simulink model "benchmark_model"  (R2021a)
settings: Solver=ode1  StartTime=0.0  StopTime=Tend  FixedStep=0.0001  MaxStep=0.1  MinStep=0.0001  AbsTol=0.01  EnableMultiTasking=on
undefined symbols (not defined in the file): A1, A2, AL, AM0, AREA, BORE, C_EGR, c_f, c_T, CAIR, cCO, cCO2, cH2, cH2O, cHC, cN2, CO, CO2, cO2, DEN0, DiscIntNeverNeededParam, EGR_dia, EGR_sk, EX_AREA, EX_M_AR, EXO, FD0, FOM, FR0, FR_C1, FR_C2, FR_C3, FR_C4, FR_C5, H2, H2O, HC, INC, INO, KET, Kex, Kh, MAS0, MCh, MHC, MN2, MO2, MOLcylT, N2, O2, PR0, R150, Rabs, SPEC, TBORE, Th_HC, Th_knock, THEX, THIN, TM0 ... (+9)
libraries: pid_lib x1
(part 5 of 6)

== system benchmark_model/ENGINE/engine_s/cylinders/cyl3/cyl/frame/Init_cyl_gas/capture_cyl_state ==
  cyl_gas : Inport
  Trigger : TriggerPort  VariantControl=(inherit)
  Add : Sum  Inputs=++++
  C+O2->CO2 : Constant  Value=4.19*97200.0
  CO+1/2O2->CO2 : Constant  Value=4.19*29620.0
  H+1/2O2->H2O : Constant  Value=4.19*57750.0
  H+1/2O2->H2O1 : Constant  Value=4.19*57750.0
  H/C : Constant  Value=y/2
  Product : Product  RndMeth=Zero
  Product1 : Product  RndMeth=Zero
  Product2 : Product  RndMeth=Zero
  Product3 : Product  Inputs=3  RndMeth=Zero
  Saturation : Saturate  UpperLimit=22  LowerLimit=6
  Selector1 : Selector  InputPortWidth=7  IndexOptions=Index vector (dialog)  Indices=[3]  OutputSizes=[(-2)]
  Selector2 : Selector  InputPortWidth=7  IndexOptions=Index vector (dialog)  Indices=[5]  OutputSizes=[(-2)]
  Selector3 : Selector  InputPortWidth=7  IndexOptions=Index vector (dialog)  Indices=[1]  OutputSizes=[(-2)]
  Selector4 : Selector  InputPortWidth=7  IndexOptions=Index vector (dialog)  Indices=[1]  OutputSizes=[(-2)]
  Subtract : Sum  Inputs=-+
  burnt_compsition : Subsystem
  cal_af : Subsystem
  Qmax : Outport
  b_comp : Outport  Port=2  InitialOutput=[0;0;0;0;0;0;0]
  init_gas : Outport  Port=3  InitialOutput=[0;0;0;0;0;0;0]
  af : Outport  Port=4  InitialOutput=0
  wires:
  Subtract/1 -> Selector3/1, Selector2/1, Selector1/1, Selector4/1
  Add/1 -> Qmax/1
  H+1/2O2->H2O/1 -> Product2/2
  Selector2/1 -> Product2/1
  CO+1/2O2->CO2/1 -> Product1/2
  Selector1/1 -> Product1/1
  C+O2->CO2/1 -> Product/2
  burnt_compsition/1(b_comp) -> b_comp/1, Subtract/1
  cal_af/1(af) -> Saturation/1, burnt_compsition/1(af)
  cyl_gas/1 -> init_gas/1, burnt_compsition/2(mol_su), Subtract/2, cal_af/1(cyl_gas)
  Product/1 -> Add/1
  Product1/1 -> Add/2
  Product2/1 -> Add/3
  H+1/2O2->H2O1/1 -> Product3/2
  Selector3/1 -> Product3/1
  Product3/1 -> Add/4
  H/C/1 -> Product3/3
  Saturation/1 -> af/1
  Selector4/1 -> Product/1

== system benchmark_model/ENGINE/engine_s/cylinders/cyl3/cyl/frame/ratio_burnt1/mod720(u,4*pi) ==
  u : Inport
  Constant7 : Constant  Value=4*pi
  Math Function : Math  Operator=mod  SignedPower=on  SaturateOnIntegerOverflow=on
  y : Outport
  wires:
  Math Function/1 -> y/1
  u/1 -> Math Function/1
  Constant7/1 -> Math Function/2

== system benchmark_model/ENGINE/engine_s/cylinders/cyl3/cyl/frame/ratio_burnt1/murnt_ratio ==
  u : Inport
  SA : Inport  Port=2
  rps : Inport  Port=3
  KL : Inport  Port=4
  AF : Inport  Port=5
  EGR : Inport  Port=6
  VT : Inport  Port=7
  Constant2 : Constant  Value=2
  Constant6 : Constant  Value=6
  Embedded MATLAB Function : MATLAB Function  TreatAsAtomicUnit=on
  Gain1 : Gain  Gain=2
  Gain2 : Gain  Gain=180/pi
  Gain3 : Gain  Gain=pi/180
  Mux : Mux
  Phi050 DoE model : Subsystem
  q : Outport
  Q : Outport  Port=2
  wires:
  Gain3/1 -> Mux/4
  Embedded MATLAB Function/1(q) -> q/1
  SA/1 -> Gain3/1, Phi050 DoE model/3(SA)
  Mux/1 -> Embedded MATLAB Function/2(Web)
  Constant6/1 -> Mux/1
  Constant2/1 -> Mux/2
  Phi050 DoE model/1(Phi50) -> Gain1/1
  rps/1 -> Phi050 DoE model/1(N)
  KL/1 -> Phi050 DoE model/2(KL)
  VT/1 -> Gain2/1
  AF/1 -> Phi050 DoE model/5(AFR)
  Gain1/1 -> Mux/3
  EGR/1 -> Phi050 DoE model/6(EGR)
  u/1 -> Embedded MATLAB Function/1(u)
  Embedded MATLAB Function/2(Q) -> Q/1
  Gain2/1 -> Phi050 DoE model/4(VVT)

== system benchmark_model/ENGINE/engine_s/cylinders/cyl3/cyl/knock_Integral/Subsystem1/Subsystem ==
  Tu : Inport
  Constant1 : Constant  Value=FR_C3
  Divide : Product  Inputs=/*
  Math Function1 : Math  SignedPower=on  SaturateOnIntegerOverflow=on
  Saturation : Saturate  UpperLimit=inf  LowerLimit=1.0e-5
  Out1 : Outport
  wires:
  Constant1/1 -> Divide/2
  Divide/1 -> Math Function1/1
  Math Function1/1 -> Out1/1
  Tu/1 -> Saturation/1
  Saturation/1 -> Divide/1

== system benchmark_model/ENGINE/engine_s/cylinders/cyl3/cyl/knock_Integral/Subsystem1/cal_unburned_temp ==
  Pc : Inport
  Tc : Inport  Port=2
  trg_inc : Inport  Port=3
  Constant : Constant  Value=1-1/Kex
  Divide3 : Product  Inputs=*/
  Divide4 : Product
  Math Function2 : Math  Operator=pow  SignedPower=on  SaturateOnIntegerOverflow=on
  Subsystem : Subsystem
  Tu : Outport
  wires:
  Subsystem/1(Pc_inc) -> Divide3/2
  Divide3/1 -> Math Function2/1
  Math Function2/1 -> Divide4/1
  Subsystem/2(Tc_inc) -> Divide4/2
  Constant/1 -> Math Function2/2
  Divide4/1 -> Tu/1
  Tc/1 -> Subsystem/2(Tc)
  Pc/1 -> Subsystem/1(Pc), Divide3/1
  trg_inc/1 -> Subsystem/Trigger

== system benchmark_model/ENGINE/engine_s/cylinders/cyl4/cyl/Energy_Int/dvol/func_d_cylvol(u,SPEC) ==
  In1 : Inport
  Constant1 : Constant  Value=SPEC
  Embedded MATLAB Function1 : MATLAB Function  TreatAsAtomicUnit=on
  Out1 : Outport
  wires:
  Embedded MATLAB Function1/1(y) -> Out1/1
  In1/1 -> Embedded MATLAB Function1/1(u)
  Constant1/1 -> Embedded MATLAB Function1/2(SPEC)

== system benchmark_model/ENGINE/engine_s/cylinders/cyl4/cyl/frame/Init_cyl_gas/capture_cyl_state ==
  cyl_gas : Inport
  Trigger : TriggerPort  VariantControl=(inherit)
  Add : Sum  Inputs=++++
  C+O2->CO2 : Constant  Value=4.19*97200.0
  CO+1/2O2->CO2 : Constant  Value=4.19*29620.0
  H+1/2O2->H2O : Constant  Value=4.19*57750.0
  H+1/2O2->H2O1 : Constant  Value=4.19*57750.0
  H/C : Constant  Value=y/2
  Product : Product  RndMeth=Zero
  Product1 : Product  RndMeth=Zero
  Product2 : Product  RndMeth=Zero
  Product3 : Product  Inputs=3  RndMeth=Zero
  Saturation : Saturate  UpperLimit=22  LowerLimit=6
  Selector1 : Selector  InputPortWidth=7  IndexOptions=Index vector (dialog)  Indices=[3]  OutputSizes=[(-2)]
  Selector2 : Selector  InputPortWidth=7  IndexOptions=Index vector (dialog)  Indices=[5]  OutputSizes=[(-2)]
  Selector3 : Selector  InputPortWidth=7  IndexOptions=Index vector (dialog)  Indices=[1]  OutputSizes=[(-2)]
  Selector4 : Selector  InputPortWidth=7  IndexOptions=Index vector (dialog)  Indices=[1]  OutputSizes=[(-2)]
  Subtract : Sum  Inputs=-+
  burnt_compsition : Subsystem
  cal_af : Subsystem
  Qmax : Outport
  b_comp : Outport  Port=2  InitialOutput=[0;0;0;0;0;0;0]
  init_gas : Outport  Port=3  InitialOutput=[0;0;0;0;0;0;0]
  af : Outport  Port=4  InitialOutput=0
  wires:
  Selector4/1 -> Product/1
  Saturation/1 -> af/1
  H/C/1 -> Product3/3
  Product3/1 -> Add/4
  Selector3/1 -> Product3/1
  H+1/2O2->H2O1/1 -> Product3/2
  Product2/1 -> Add/3
  Product1/1 -> Add/2
  Product/1 -> Add/1
  cyl_gas/1 -> cal_af/1(cyl_gas), Subtract/2, burnt_compsition/2(mol_su), init_gas/1
  cal_af/1(af) -> burnt_compsition/1(af), Saturation/1
  burnt_compsition/1(b_comp) -> Subtract/1, b_comp/1
  C+O2->CO2/1 -> Product/2
  Selector1/1 -> Product1/1
  CO+1/2O2->CO2/1 -> Product1/2
  Selector2/1 -> Product2/1
  H+1/2O2->H2O/1 -> Product2/2
  Add/1 -> Qmax/1
  Subtract/1 -> Selector4/1, Selector1/1, Selector2/1, Selector3/1

== system benchmark_model/ENGINE/engine_s/cylinders/cyl4/cyl/frame/ratio_burnt1/mod720(u,4*pi) ==
  u : Inport
  Constant7 : Constant  Value=4*pi
  Math Function : Math  Operator=mod  SignedPower=on  SaturateOnIntegerOverflow=on
  y : Outport
  wires:
  Constant7/1 -> Math Function/2
  u/1 -> Math Function/1
  Math Function/1 -> y/1

== system benchmark_model/ENGINE/engine_s/cylinders/cyl4/cyl/frame/ratio_burnt1/murnt_ratio ==
  u : Inport
  SA : Inport  Port=2
  rps : Inport  Port=3
  KL : Inport  Port=4
  AF : Inport  Port=5
  EGR : Inport  Port=6
  VT : Inport  Port=7
  Constant2 : Constant  Value=2
  Constant6 : Constant  Value=6
  Embedded MATLAB Function : MATLAB Function  TreatAsAtomicUnit=on
  Gain1 : Gain  Gain=2
  Gain2 : Gain  Gain=180/pi
  Gain3 : Gain  Gain=pi/180
  Mux : Mux
  Phi050 DoE model : Subsystem
  q : Outport
  Q : Outport  Port=2
  wires:
  Gain2/1 -> Phi050 DoE model/4(VVT)
  Embedded MATLAB Function/2(Q) -> Q/1
  u/1 -> Embedded MATLAB Function/1(u)
  EGR/1 -> Phi050 DoE model/6(EGR)
  Gain1/1 -> Mux/3
  AF/1 -> Phi050 DoE model/5(AFR)
  VT/1 -> Gain2/1
  KL/1 -> Phi050 DoE model/2(KL)
  rps/1 -> Phi050 DoE model/1(N)
  Phi050 DoE model/1(Phi50) -> Gain1/1
  Constant2/1 -> Mux/2
  Constant6/1 -> Mux/1
  Mux/1 -> Embedded MATLAB Function/2(Web)
  SA/1 -> Phi050 DoE model/3(SA), Gain3/1
  Embedded MATLAB Function/1(q) -> q/1
  Gain3/1 -> Mux/4

== system benchmark_model/ENGINE/engine_s/cylinders/cyl4/cyl/knock_Integral/Subsystem1/Subsystem ==
  Tu : Inport
  Constant1 : Constant  Value=FR_C3
  Divide : Product  Inputs=/*
  Math Function1 : Math  SignedPower=on  SaturateOnIntegerOverflow=on
  Saturation : Saturate  UpperLimit=inf  LowerLimit=1.0e-5
  Out1 : Outport
  wires:
  Saturation/1 -> Divide/1
  Tu/1 -> Saturation/1
  Math Function1/1 -> Out1/1
  Divide/1 -> Math Function1/1
  Constant1/1 -> Divide/2

== system benchmark_model/ENGINE/engine_s/cylinders/cyl4/cyl/knock_Integral/Subsystem1/cal_unburned_temp ==
  Pc : Inport
  Tc : Inport  Port=2
  trg_inc : Inport  Port=3
  Constant : Constant  Value=1-1/Kex
  Divide3 : Product  Inputs=*/
  Divide4 : Product
  Math Function2 : Math  Operator=pow  SignedPower=on  SaturateOnIntegerOverflow=on
  Subsystem : Subsystem
  Tu : Outport
  wires:
  trg_inc/1 -> Subsystem/Trigger
  Pc/1 -> Divide3/1, Subsystem/1(Pc)
  Tc/1 -> Subsystem/2(Tc)
  Divide4/1 -> Tu/1
  Constant/1 -> Math Function2/2
  Subsystem/2(Tc_inc) -> Divide4/2
  Math Function2/1 -> Divide4/1
  Divide3/1 -> Math Function2/1
  Subsystem/1(Pc_inc) -> Divide3/2

== system benchmark_model/ENGINE/engine_s/cylinders/cyl1/cyl/frame/Init_cyl_gas/capture_cyl_state/burnt_compsition ==
  af : Inport
  mol_su : Inport  Port=2
  C : Constant  Value=WOM
  C1 : Constant  Value=WOM
  Dot Product : DotProduct  InputSameDT=on  OutDataTypeStr=Inherit: Inherit via internal rule
  Dot Product2 : DotProduct  InputSameDT=on  OutDataTypeStr=Inherit: Inherit via internal rule
  Mux : Mux  Inputs=7
  Product1 : Product  RndMeth=Zero
  Product2 : Product  Inputs=/*  RndMeth=Zero
  Saturation : Saturate  UpperLimit=22  LowerLimit=6
  Subsystem : Subsystem
  table_CO : Lookup  InputValues=AL  Table=[CO]*1.0e-2
  table_CO2 : Lookup  InputValues=AL  Table=[CO2]*1.0e-2
  table_H2 : Lookup  InputValues=AL  Table=[H2]*1.0e-2
  table_H2O : Lookup  InputValues=AL  Table=[H2O]*1.0e-2
  table_HC : Lookup  InputValues=AL  Table=[HC]*1.0e-6
  table_N2 : Lookup  InputValues=AL  Table=[N2]*1.0e-2
  table_O2 : Lookup  InputValues=AL  Table=[O2]*1.0e-2
  b_comp : Outport
  wires:
  Product2/1 -> Product1/2
  Product1/1 -> Subsystem/2(burnt)
  C/1 -> Dot Product/2
  table_HC/1 -> Mux/1
  table_N2/1 -> Mux/7
  table_CO2/1 -> Mux/2
  table_CO/1 -> Mux/3
  table_O2/1 -> Mux/4
  table_H2/1 -> Mux/5
  table_H2O/1 -> Mux/6
  af/1 -> Saturation/1, Subsystem/1(af)
  Mux/1 -> Product1/1, Dot Product/1
  Saturation/1 -> table_HC/1, table_CO2/1, table_CO/1, table_O2/1, table_H2/1, table_H2O/1, table_N2/1
  mol_su/1 -> Subsystem/3(unburnt), Dot Product2/2
  Subsystem/1(Out1) -> b_comp/1
  C1/1 -> Dot Product2/1
  Dot Product/1 -> Product2/1
  Dot Product2/1 -> Product2/2

== system benchmark_model/ENGINE/engine_s/cylinders/cyl1/cyl/frame/Init_cyl_gas/capture_cyl_state/cal_af ==
  cyl_gas : Inport
  Constant2 : Constant  Value=[0,MO2,MO2/2,MO2,0,MO2/2,MN2]
  Constant3 : Constant  Value=[1,1,1,0,0,0,0]
  Divide : Product  Inputs=/*
  Dot Product : DotProduct  InputSameDT=on  OutDataTypeStr=Inherit: Inherit via internal rule
  Dot Product2 : DotProduct  InputSameDT=on  OutDataTypeStr=Inherit: Inherit via internal rule
  Gain : Gain  Gain=MHC
  af : Outport
  wires:
  Gain/1 -> Divide/1
  Divide/1 -> af/1
  Constant3/1 -> Dot Product/2
  Dot Product/1 -> Gain/1
  cyl_gas/1 -> Dot Product/1, Dot Product2/1
  Dot Product2/1 -> Divide/2
  Constant2/1 -> Dot Product2/2

== system benchmark_model/ENGINE/engine_s/cylinders/cyl1/cyl/frame/ratio_burnt1/murnt_ratio/Phi050 DoE model ==
  N : Inport
  KL : Inport  Port=2
  SA : Inport  Port=3
  VVT : Inport  Port=4
  AFR : Inport  Port=5
  EGR : Inport  Port=6
  0 .. 1 : Saturate  UpperLimit=0.9  LowerLimit=0  ZeroCross=off
      settings: AttributesFormatString=%<LowerLimit> .. %<UpperLimit>
  Fcn : Fcn  Expr=C_EGR/(1-u)
  Product : Product
  Subsystem : Subsystem
  Phi50 : Outport
  wires:
  N/1 -> Subsystem/1(N)
  KL/1 -> Subsystem/2(KL)
  SA/1 -> Subsystem/3(SA)
  VVT/1 -> Subsystem/4(VVT)
  Subsystem/1(Phi50) -> Phi50/1
  EGR/1 -> 0 .. 1/1
  0 .. 1/1 -> Fcn/1
  AFR/1 -> Product/1
  Fcn/1 -> Product/2
  Product/1 -> Subsystem/5(AFR)

== system benchmark_model/ENGINE/engine_s/cylinders/cyl1/cyl/knock_Integral/Subsystem1/cal_unburned_temp/Subsystem ==
  Pc : Inport
  Tc : Inport  Port=2
  Trigger : TriggerPort  VariantControl=(inherit)
  Pc_inc : Outport  InitialOutput=[PR0]
  Tc_inc : Outport  Port=2  InitialOutput=[TM0]
  wires:
  Tc/1 -> Tc_inc/1
  Pc/1 -> Pc_inc/1

== system benchmark_model/ENGINE/engine_s/cylinders/cyl2/cyl/frame/Init_cyl_gas/capture_cyl_state/burnt_compsition ==
  af : Inport
  mol_su : Inport  Port=2
  C : Constant  Value=WOM
  C1 : Constant  Value=WOM
  Dot Product : DotProduct  InputSameDT=on  OutDataTypeStr=Inherit: Inherit via internal rule
  Dot Product2 : DotProduct  InputSameDT=on  OutDataTypeStr=Inherit: Inherit via internal rule
  Mux : Mux  Inputs=7
  Product1 : Product  RndMeth=Zero
  Product2 : Product  Inputs=/*  RndMeth=Zero
  Saturation : Saturate  UpperLimit=22  LowerLimit=6
  Subsystem : Subsystem
  table_CO : Lookup  InputValues=AL  Table=[CO]*1.0e-2
  table_CO2 : Lookup  InputValues=AL  Table=[CO2]*1.0e-2
  table_H2 : Lookup  InputValues=AL  Table=[H2]*1.0e-2
  table_H2O : Lookup  InputValues=AL  Table=[H2O]*1.0e-2
  table_HC : Lookup  InputValues=AL  Table=[HC]*1.0e-6
  table_N2 : Lookup  InputValues=AL  Table=[N2]*1.0e-2
  table_O2 : Lookup  InputValues=AL  Table=[O2]*1.0e-2
  b_comp : Outport
  wires:
  Dot Product2/1 -> Product2/2
  Dot Product/1 -> Product2/1
  C1/1 -> Dot Product2/1
  Subsystem/1(Out1) -> b_comp/1
  mol_su/1 -> Dot Product2/2, Subsystem/3(unburnt)
  Saturation/1 -> table_N2/1, table_H2O/1, table_H2/1, table_O2/1, table_CO/1, table_CO2/1, table_HC/1
  Mux/1 -> Dot Product/1, Product1/1
  af/1 -> Subsystem/1(af), Saturation/1
  table_H2O/1 -> Mux/6
  table_H2/1 -> Mux/5
  table_O2/1 -> Mux/4
  table_CO/1 -> Mux/3
  table_CO2/1 -> Mux/2
  table_N2/1 -> Mux/7
  table_HC/1 -> Mux/1
  C/1 -> Dot Product/2
  Product1/1 -> Subsystem/2(burnt)
  Product2/1 -> Product1/2

== system benchmark_model/ENGINE/engine_s/cylinders/cyl2/cyl/frame/Init_cyl_gas/capture_cyl_state/cal_af ==
  cyl_gas : Inport
  Constant2 : Constant  Value=[0,MO2,MO2/2,MO2,0,MO2/2,MN2]
  Constant3 : Constant  Value=[1,1,1,0,0,0,0]
  Divide : Product  Inputs=/*
  Dot Product : DotProduct  InputSameDT=on  OutDataTypeStr=Inherit: Inherit via internal rule
  Dot Product2 : DotProduct  InputSameDT=on  OutDataTypeStr=Inherit: Inherit via internal rule
  Gain : Gain  Gain=MHC
  af : Outport
  wires:
  Constant2/1 -> Dot Product2/2
  Dot Product2/1 -> Divide/2
  cyl_gas/1 -> Dot Product2/1, Dot Product/1
  Dot Product/1 -> Gain/1
  Constant3/1 -> Dot Product/2
  Divide/1 -> af/1
  Gain/1 -> Divide/1

== system benchmark_model/ENGINE/engine_s/cylinders/cyl2/cyl/frame/ratio_burnt1/murnt_ratio/Phi050 DoE model ==
  N : Inport
  KL : Inport  Port=2
  SA : Inport  Port=3
  VVT : Inport  Port=4
  AFR : Inport  Port=5
  EGR : Inport  Port=6
  0 .. 1 : Saturate  UpperLimit=0.9  LowerLimit=0  ZeroCross=off
      settings: AttributesFormatString=%<LowerLimit> .. %<UpperLimit>
  Fcn : Fcn  Expr=C_EGR/(1-u)
  Product : Product
  Subsystem : Subsystem
  Phi50 : Outport
  wires:
  Product/1 -> Subsystem/5(AFR)
  Fcn/1 -> Product/2
  AFR/1 -> Product/1
  0 .. 1/1 -> Fcn/1
  EGR/1 -> 0 .. 1/1
  Subsystem/1(Phi50) -> Phi50/1
  VVT/1 -> Subsystem/4(VVT)
  SA/1 -> Subsystem/3(SA)
  KL/1 -> Subsystem/2(KL)
  N/1 -> Subsystem/1(N)

== system benchmark_model/ENGINE/engine_s/cylinders/cyl2/cyl/knock_Integral/Subsystem1/cal_unburned_temp/Subsystem ==
  Pc : Inport
  Tc : Inport  Port=2
  Trigger : TriggerPort  VariantControl=(inherit)
  Pc_inc : Outport  InitialOutput=[PR0]
  Tc_inc : Outport  Port=2  InitialOutput=[TM0]
  wires:
  Pc/1 -> Pc_inc/1
  Tc/1 -> Tc_inc/1

== system benchmark_model/ENGINE/engine_s/cylinders/cyl3/cyl/frame/Init_cyl_gas/capture_cyl_state/burnt_compsition ==
  af : Inport
  mol_su : Inport  Port=2
  C : Constant  Value=WOM
  C1 : Constant  Value=WOM
  Dot Product : DotProduct  InputSameDT=on  OutDataTypeStr=Inherit: Inherit via internal rule
  Dot Product2 : DotProduct  InputSameDT=on  OutDataTypeStr=Inherit: Inherit via internal rule
  Mux : Mux  Inputs=7
  Product1 : Product  RndMeth=Zero
  Product2 : Product  Inputs=/*  RndMeth=Zero
  Saturation : Saturate  UpperLimit=22  LowerLimit=6
  Subsystem : Subsystem
  table_CO : Lookup  InputValues=AL  Table=[CO]*1.0e-2
  table_CO2 : Lookup  InputValues=AL  Table=[CO2]*1.0e-2
  table_H2 : Lookup  InputValues=AL  Table=[H2]*1.0e-2
  table_H2O : Lookup  InputValues=AL  Table=[H2O]*1.0e-2
  table_HC : Lookup  InputValues=AL  Table=[HC]*1.0e-6
  table_N2 : Lookup  InputValues=AL  Table=[N2]*1.0e-2
  table_O2 : Lookup  InputValues=AL  Table=[O2]*1.0e-2
  b_comp : Outport
  wires:
  Product2/1 -> Product1/2
  Product1/1 -> Subsystem/2(burnt)
  C/1 -> Dot Product/2
  table_HC/1 -> Mux/1
  table_N2/1 -> Mux/7
  table_CO2/1 -> Mux/2
  table_CO/1 -> Mux/3
  table_O2/1 -> Mux/4
  table_H2/1 -> Mux/5
  table_H2O/1 -> Mux/6
  af/1 -> Saturation/1, Subsystem/1(af)
  Mux/1 -> Product1/1, Dot Product/1
  Saturation/1 -> table_HC/1, table_CO2/1, table_CO/1, table_O2/1, table_H2/1, table_H2O/1, table_N2/1
  mol_su/1 -> Subsystem/3(unburnt), Dot Product2/2
  Subsystem/1(Out1) -> b_comp/1
  C1/1 -> Dot Product2/1
  Dot Product/1 -> Product2/1
  Dot Product2/1 -> Product2/2

== system benchmark_model/ENGINE/engine_s/cylinders/cyl3/cyl/frame/Init_cyl_gas/capture_cyl_state/cal_af ==
  cyl_gas : Inport
  Constant2 : Constant  Value=[0,MO2,MO2/2,MO2,0,MO2/2,MN2]
  Constant3 : Constant  Value=[1,1,1,0,0,0,0]
  Divide : Product  Inputs=/*
  Dot Product : DotProduct  InputSameDT=on  OutDataTypeStr=Inherit: Inherit via internal rule
  Dot Product2 : DotProduct  InputSameDT=on  OutDataTypeStr=Inherit: Inherit via internal rule
  Gain : Gain  Gain=MHC
  af : Outport
  wires:
  Gain/1 -> Divide/1
  Divide/1 -> af/1
  Constant3/1 -> Dot Product/2
  Dot Product/1 -> Gain/1
  cyl_gas/1 -> Dot Product/1, Dot Product2/1
  Dot Product2/1 -> Divide/2
  Constant2/1 -> Dot Product2/2

== system benchmark_model/ENGINE/engine_s/cylinders/cyl3/cyl/frame/ratio_burnt1/murnt_ratio/Phi050 DoE model ==
  N : Inport
  KL : Inport  Port=2
  SA : Inport  Port=3
  VVT : Inport  Port=4
  AFR : Inport  Port=5
  EGR : Inport  Port=6
  0 .. 1 : Saturate  UpperLimit=0.9  LowerLimit=0  ZeroCross=off
      settings: AttributesFormatString=%<LowerLimit> .. %<UpperLimit>
  Fcn : Fcn  Expr=C_EGR/(1-u)
  Product : Product
  Subsystem : Subsystem
  Phi50 : Outport
  wires:
  N/1 -> Subsystem/1(N)
  KL/1 -> Subsystem/2(KL)
  SA/1 -> Subsystem/3(SA)
  VVT/1 -> Subsystem/4(VVT)
  Subsystem/1(Phi50) -> Phi50/1
  EGR/1 -> 0 .. 1/1
  0 .. 1/1 -> Fcn/1
  AFR/1 -> Product/1
  Fcn/1 -> Product/2
  Product/1 -> Subsystem/5(AFR)

== system benchmark_model/ENGINE/engine_s/cylinders/cyl3/cyl/knock_Integral/Subsystem1/cal_unburned_temp/Subsystem ==
  Pc : Inport
  Tc : Inport  Port=2
  Trigger : TriggerPort  VariantControl=(inherit)
  Pc_inc : Outport  InitialOutput=[PR0]
  Tc_inc : Outport  Port=2  InitialOutput=[TM0]
  wires:
  Tc/1 -> Tc_inc/1
  Pc/1 -> Pc_inc/1

== system benchmark_model/ENGINE/engine_s/cylinders/cyl4/cyl/frame/Init_cyl_gas/capture_cyl_state/burnt_compsition ==
  af : Inport
  mol_su : Inport  Port=2
  C : Constant  Value=WOM
  C1 : Constant  Value=WOM
  Dot Product : DotProduct  InputSameDT=on  OutDataTypeStr=Inherit: Inherit via internal rule
  Dot Product2 : DotProduct  InputSameDT=on  OutDataTypeStr=Inherit: Inherit via internal rule
  Mux : Mux  Inputs=7
  Product1 : Product  RndMeth=Zero
  Product2 : Product  Inputs=/*  RndMeth=Zero
  Saturation : Saturate  UpperLimit=22  LowerLimit=6
  Subsystem : Subsystem
  table_CO : Lookup  InputValues=AL  Table=[CO]*1.0e-2
  table_CO2 : Lookup  InputValues=AL  Table=[CO2]*1.0e-2
  table_H2 : Lookup  InputValues=AL  Table=[H2]*1.0e-2
  table_H2O : Lookup  InputValues=AL  Table=[H2O]*1.0e-2
  table_HC : Lookup  InputValues=AL  Table=[HC]*1.0e-6
  table_N2 : Lookup  InputValues=AL  Table=[N2]*1.0e-2
  table_O2 : Lookup  InputValues=AL  Table=[O2]*1.0e-2
  b_comp : Outport
  wires:
  Dot Product2/1 -> Product2/2
  Dot Product/1 -> Product2/1
  C1/1 -> Dot Product2/1
  Subsystem/1(Out1) -> b_comp/1
  mol_su/1 -> Dot Product2/2, Subsystem/3(unburnt)
  Saturation/1 -> table_N2/1, table_H2O/1, table_H2/1, table_O2/1, table_CO/1, table_CO2/1, table_HC/1
  Mux/1 -> Dot Product/1, Product1/1
  af/1 -> Subsystem/1(af), Saturation/1
  table_H2O/1 -> Mux/6
  table_H2/1 -> Mux/5
  table_O2/1 -> Mux/4
  table_CO/1 -> Mux/3
  table_CO2/1 -> Mux/2
  table_N2/1 -> Mux/7
  table_HC/1 -> Mux/1
  C/1 -> Dot Product/2
  Product1/1 -> Subsystem/2(burnt)
  Product2/1 -> Product1/2

== system benchmark_model/ENGINE/engine_s/cylinders/cyl4/cyl/frame/Init_cyl_gas/capture_cyl_state/cal_af ==
  cyl_gas : Inport
  Constant2 : Constant  Value=[0,MO2,MO2/2,MO2,0,MO2/2,MN2]
  Constant3 : Constant  Value=[1,1,1,0,0,0,0]
  Divide : Product  Inputs=/*
  Dot Product : DotProduct  InputSameDT=on  OutDataTypeStr=Inherit: Inherit via internal rule
  Dot Product2 : DotProduct  InputSameDT=on  OutDataTypeStr=Inherit: Inherit via internal rule
  Gain : Gain  Gain=MHC
  af : Outport
  wires:
  Constant2/1 -> Dot Product2/2
  Dot Product2/1 -> Divide/2
  cyl_gas/1 -> Dot Product2/1, Dot Product/1
  Dot Product/1 -> Gain/1
  Constant3/1 -> Dot Product/2
  Divide/1 -> af/1
  Gain/1 -> Divide/1

== system benchmark_model/ENGINE/engine_s/cylinders/cyl4/cyl/frame/ratio_burnt1/murnt_ratio/Phi050 DoE model ==
  N : Inport
  KL : Inport  Port=2
  SA : Inport  Port=3
  VVT : Inport  Port=4
  AFR : Inport  Port=5
  EGR : Inport  Port=6
  0 .. 1 : Saturate  UpperLimit=0.9  LowerLimit=0  ZeroCross=off
      settings: AttributesFormatString=%<LowerLimit> .. %<UpperLimit>
  Fcn : Fcn  Expr=C_EGR/(1-u)
  Product : Product
  Subsystem : Subsystem
  Phi50 : Outport
  wires:
  Product/1 -> Subsystem/5(AFR)
  Fcn/1 -> Product/2
  AFR/1 -> Product/1
  0 .. 1/1 -> Fcn/1
  EGR/1 -> 0 .. 1/1
  Subsystem/1(Phi50) -> Phi50/1
  VVT/1 -> Subsystem/4(VVT)
  SA/1 -> Subsystem/3(SA)
  KL/1 -> Subsystem/2(KL)
  N/1 -> Subsystem/1(N)

== system benchmark_model/ENGINE/engine_s/cylinders/cyl4/cyl/knock_Integral/Subsystem1/cal_unburned_temp/Subsystem ==
  Pc : Inport
  Tc : Inport  Port=2
  Trigger : TriggerPort  VariantControl=(inherit)
  Pc_inc : Outport  InitialOutput=[PR0]
  Tc_inc : Outport  Port=2  InitialOutput=[TM0]
  wires:
  Pc/1 -> Pc_inc/1
  Tc/1 -> Tc_inc/1

== system benchmark_model/ENGINE/engine_s/cylinders/cyl1/cyl/frame/Init_cyl_gas/capture_cyl_state/burnt_compsition/Subsystem ==
  af : Inport
  burnt : Inport  Port=2
  unburnt : Inport  Port=3
  C1 : Constant  Value=6
  C2 : Constant  Value=22
  Logical Operator : Logic  AllPortsSameDT=off  OutDataTypeStr=boolean
  Relational Operator : RelationalOperator  OutDataTypeStr=boolean  RndMeth=Nearest
  Relational Operator1 : RelationalOperator  Operator=<=  OutDataTypeStr=boolean  RndMeth=Nearest
  Switch : Switch  Threshold=0.5
  Out1 : Outport
  wires:
  Logical Operator/1 -> Switch/2
  Relational Operator/1 -> Logical Operator/1
  Relational Operator1/1 -> Logical Operator/2
  C2/1 -> Relational Operator1/2
  C1/1 -> Relational Operator/2
  af/1 -> Relational Operator1/1, Relational Operator/1
  burnt/1 -> Switch/1
  Switch/1 -> Out1/1
  unburnt/1 -> Switch/3

== system benchmark_model/ENGINE/engine_s/cylinders/cyl1/cyl/frame/ratio_burnt1/murnt_ratio/Phi050 DoE model/Subsystem ==
  note: SAmin changed from 0 to -15deg, PS1303131400
      |
      | N=((2*N-6599)./(5401));
      | KL=((2*KL-104.17)./(71.89));
      | LA=((2*LA-1.801)./(0.235));
      | VVT=((2*VVT-46.18)./(46.18));
      | SP=((2*SA-49)./(49));
      | EG=C02/interp(AL,CO2,14.5);
      | phi50-spark=exp(3.6636+0.16333.*N-0.2286.*KL+0.067945.*LA+0.058803.*VVT-0.1392.*SP+0.30732.*SP.^2-0.3238.*N.*SP);
  N : Inport
  KL : Inport  Port=2
  SA : Inport  Port=3
  VVT : Inport  Port=4
  AFR : Inport  Port=5
  ->% : Gain  Gain=100
  0 .. 50 : Saturate  UpperLimit=50  LowerLimit=-15  ZeroCross=off
      settings: AttributesFormatString=%<LowerLimit> .. %<UpperLimit>
  0 ..1 : Saturate  UpperLimit=1.013*0+2.0  LowerLimit=.803  ZeroCross=off
      settings: AttributesFormatString=%<LowerLimit> .. %<UpperLimit>
  0 ..50 : Saturate  UpperLimit=50  LowerLimit=0  ZeroCross=off
      settings: AttributesFormatString=%<LowerLimit> .. %<UpperLimit>
  10 .. 100 : Saturate  UpperLimit=88.03  LowerLimit=16.64  ZeroCross=off
      settings: AttributesFormatString=%<LowerLimit> .. %<UpperLimit>
  600 .. 6000 : Saturate  UpperLimit=6000  LowerLimit=599  ZeroCross=off
      settings: AttributesFormatString=%<LowerLimit> .. %<UpperLimit>
  AFR->lambda : Gain  Gain=1/14.5
  DoE-Model PRESS 3.75 : Fcn  Expr=exp(3.6636+0.16333*u(1)-0.2286*u(2)+0.067945*u(3)+0.058803*u(4)-0.1392*u(5)+0.30732*u(5)^2-0.3238*u(1)*u(5))
  Fcn1 : Fcn  Expr=2*(u-599)/(6000-599)-1
      settings: AttributesFormatString=%<Expr>
  Fcn4 : Fcn  Expr=2*(u-16.64)/(88.03-16.64)-1
      settings: AttributesFormatString=%<Expr>
  Fcn5 : Fcn  Expr=2*(u-0)/(49-0)-1
      settings: AttributesFormatString=%<Expr>
  Fcn6 : Fcn  Expr=2*(u-40)/(46.18-0)-1
      settings: AttributesFormatString=%<Expr>
  Fcn7 : Fcn  Expr=2*(u-0.803)/(1.013-0.803)-1
      settings: AttributesFormatString=%<Expr>
  Mx1 : Mux  Inputs=5
  deg->SI : Gain  Gain=pi/180
  rad->deg : Gain
  Phi50 : Outport
  wires:
  deg->SI/1 -> Phi50/1
  Fcn5/1 -> Mx1/5
  DoE-Model PRESS 3.75/1 -> deg->SI/1
  Fcn7/1 -> Mx1/3
  0 ..1/1 -> Fcn7/1
  AFR/1 -> AFR->lambda/1
  AFR->lambda/1 -> 0 ..1/1  "VVTdeg"
  Fcn6/1 -> Mx1/4
  Fcn4/1 -> Mx1/2
  Fcn1/1 -> Mx1/1
  0 ..50/1 -> Fcn6/1
  SA/1 -> 0 .. 50/1
  0 .. 50/1 -> Fcn5/1
  Mx1/1 -> DoE-Model PRESS 3.75/1
  VVT/1 -> rad->deg/1
  KL/1 -> ->%/1
  N/1 -> 600 .. 6000/1
  ->%/1 -> 10 .. 100/1
  10 .. 100/1 -> Fcn4/1  "KL"
  600 .. 6000/1 -> Fcn1/1  "N"
  rad->deg/1 -> 0 ..50/1  "VVTdeg"

== system benchmark_model/ENGINE/engine_s/cylinders/cyl2/cyl/frame/Init_cyl_gas/capture_cyl_state/burnt_compsition/Subsystem ==
  af : Inport
  burnt : Inport  Port=2
  unburnt : Inport  Port=3
  C1 : Constant  Value=6
  C2 : Constant  Value=22
  Logical Operator : Logic  AllPortsSameDT=off  OutDataTypeStr=boolean
  Relational Operator : RelationalOperator  OutDataTypeStr=boolean  RndMeth=Nearest
  Relational Operator1 : RelationalOperator  Operator=<=  OutDataTypeStr=boolean  RndMeth=Nearest
  Switch : Switch  Threshold=0.5
  Out1 : Outport
  wires:
  unburnt/1 -> Switch/3
  Switch/1 -> Out1/1
  burnt/1 -> Switch/1
  af/1 -> Relational Operator/1, Relational Operator1/1
  C1/1 -> Relational Operator/2
  C2/1 -> Relational Operator1/2
  Relational Operator1/1 -> Logical Operator/2
  Relational Operator/1 -> Logical Operator/1
  Logical Operator/1 -> Switch/2

== system benchmark_model/ENGINE/engine_s/cylinders/cyl2/cyl/frame/ratio_burnt1/murnt_ratio/Phi050 DoE model/Subsystem ==
  note: SAmin changed from 0 to -15deg, PS1303131400
      |
      | N=((2*N-6599)./(5401));
      | KL=((2*KL-104.17)./(71.89));
      | LA=((2*LA-1.801)./(0.235));
      | VVT=((2*VVT-46.18)./(46.18));
      | SP=((2*SA-49)./(49));
      | EG=C02/interp(AL,CO2,14.5);
      | phi50-spark=exp(3.6636+0.16333.*N-0.2286.*KL+0.067945.*LA+0.058803.*VVT-0.1392.*SP+0.30732.*SP.^2-0.3238.*N.*SP);
  N : Inport
  KL : Inport  Port=2
  SA : Inport  Port=3
  VVT : Inport  Port=4
  AFR : Inport  Port=5
  ->% : Gain  Gain=100
  0 .. 50 : Saturate  UpperLimit=50  LowerLimit=-15  ZeroCross=off
      settings: AttributesFormatString=%<LowerLimit> .. %<UpperLimit>
  0 ..1 : Saturate  UpperLimit=1.013*0+2.0  LowerLimit=.803  ZeroCross=off
      settings: AttributesFormatString=%<LowerLimit> .. %<UpperLimit>
  0 ..50 : Saturate  UpperLimit=50  LowerLimit=0  ZeroCross=off
      settings: AttributesFormatString=%<LowerLimit> .. %<UpperLimit>
  10 .. 100 : Saturate  UpperLimit=88.03  LowerLimit=16.64  ZeroCross=off
      settings: AttributesFormatString=%<LowerLimit> .. %<UpperLimit>
  600 .. 6000 : Saturate  UpperLimit=6000  LowerLimit=599  ZeroCross=off
      settings: AttributesFormatString=%<LowerLimit> .. %<UpperLimit>
  AFR->lambda : Gain  Gain=1/14.5
  DoE-Model PRESS 3.75 : Fcn  Expr=exp(3.6636+0.16333*u(1)-0.2286*u(2)+0.067945*u(3)+0.058803*u(4)-0.1392*u(5)+0.30732*u(5)^2-0.3238*u(1)*u(5))
  Fcn1 : Fcn  Expr=2*(u-599)/(6000-599)-1
      settings: AttributesFormatString=%<Expr>
  Fcn4 : Fcn  Expr=2*(u-16.64)/(88.03-16.64)-1
      settings: AttributesFormatString=%<Expr>
  Fcn5 : Fcn  Expr=2*(u-0)/(49-0)-1
      settings: AttributesFormatString=%<Expr>
  Fcn6 : Fcn  Expr=2*(u-40)/(46.18-0)-1
      settings: AttributesFormatString=%<Expr>
  Fcn7 : Fcn  Expr=2*(u-0.803)/(1.013-0.803)-1
      settings: AttributesFormatString=%<Expr>
  Mx1 : Mux  Inputs=5
  deg->SI : Gain  Gain=pi/180
  rad->deg : Gain
  Phi50 : Outport
  wires:
  rad->deg/1 -> 0 ..50/1  "VVTdeg"
  600 .. 6000/1 -> Fcn1/1  "N"
  10 .. 100/1 -> Fcn4/1  "KL"
  ->%/1 -> 10 .. 100/1
  N/1 -> 600 .. 6000/1
  KL/1 -> ->%/1
  VVT/1 -> rad->deg/1
  Mx1/1 -> DoE-Model PRESS 3.75/1
  0 .. 50/1 -> Fcn5/1
  SA/1 -> 0 .. 50/1
  0 ..50/1 -> Fcn6/1
  Fcn1/1 -> Mx1/1
  Fcn4/1 -> Mx1/2
  Fcn6/1 -> Mx1/4
  AFR->lambda/1 -> 0 ..1/1  "VVTdeg"
  AFR/1 -> AFR->lambda/1
  0 ..1/1 -> Fcn7/1
  Fcn7/1 -> Mx1/3
  DoE-Model PRESS 3.75/1 -> deg->SI/1
  Fcn5/1 -> Mx1/5
  deg->SI/1 -> Phi50/1

== system benchmark_model/ENGINE/engine_s/cylinders/cyl3/cyl/frame/Init_cyl_gas/capture_cyl_state/burnt_compsition/Subsystem ==
  af : Inport
  burnt : Inport  Port=2
  unburnt : Inport  Port=3
  C1 : Constant  Value=6
  C2 : Constant  Value=22
  Logical Operator : Logic  AllPortsSameDT=off  OutDataTypeStr=boolean
  Relational Operator : RelationalOperator  OutDataTypeStr=boolean  RndMeth=Nearest
  Relational Operator1 : RelationalOperator  Operator=<=  OutDataTypeStr=boolean  RndMeth=Nearest
  Switch : Switch  Threshold=0.5
  Out1 : Outport
  wires:
  Logical Operator/1 -> Switch/2
  Relational Operator/1 -> Logical Operator/1
  Relational Operator1/1 -> Logical Operator/2
  C2/1 -> Relational Operator1/2
  C1/1 -> Relational Operator/2
  af/1 -> Relational Operator1/1, Relational Operator/1
  burnt/1 -> Switch/1
  Switch/1 -> Out1/1
  unburnt/1 -> Switch/3

== system benchmark_model/ENGINE/engine_s/cylinders/cyl3/cyl/frame/ratio_burnt1/murnt_ratio/Phi050 DoE model/Subsystem ==
  note: SAmin changed from 0 to -15deg, PS1303131400
      |
      | N=((2*N-6599)./(5401));
      | KL=((2*KL-104.17)./(71.89));
      | LA=((2*LA-1.801)./(0.235));
      | VVT=((2*VVT-46.18)./(46.18));
      | SP=((2*SA-49)./(49));
      | EG=C02/interp(AL,CO2,14.5);
      | phi50-spark=exp(3.6636+0.16333.*N-0.2286.*KL+0.067945.*LA+0.058803.*VVT-0.1392.*SP+0.30732.*SP.^2-0.3238.*N.*SP);
  N : Inport
  KL : Inport  Port=2
  SA : Inport  Port=3
  VVT : Inport  Port=4
  AFR : Inport  Port=5
  ->% : Gain  Gain=100
  0 .. 50 : Saturate  UpperLimit=50  LowerLimit=-15  ZeroCross=off
      settings: AttributesFormatString=%<LowerLimit> .. %<UpperLimit>
  0 ..1 : Saturate  UpperLimit=1.013*0+2.0  LowerLimit=.803  ZeroCross=off
      settings: AttributesFormatString=%<LowerLimit> .. %<UpperLimit>
  0 ..50 : Saturate  UpperLimit=50  LowerLimit=0  ZeroCross=off
      settings: AttributesFormatString=%<LowerLimit> .. %<UpperLimit>
  10 .. 100 : Saturate  UpperLimit=88.03  LowerLimit=16.64  ZeroCross=off
      settings: AttributesFormatString=%<LowerLimit> .. %<UpperLimit>
  600 .. 6000 : Saturate  UpperLimit=6000  LowerLimit=599  ZeroCross=off
      settings: AttributesFormatString=%<LowerLimit> .. %<UpperLimit>
  AFR->lambda : Gain  Gain=1/14.5
  DoE-Model PRESS 3.75 : Fcn  Expr=exp(3.6636+0.16333*u(1)-0.2286*u(2)+0.067945*u(3)+0.058803*u(4)-0.1392*u(5)+0.30732*u(5)^2-0.3238*u(1)*u(5))
  Fcn1 : Fcn  Expr=2*(u-599)/(6000-599)-1
      settings: AttributesFormatString=%<Expr>
  Fcn4 : Fcn  Expr=2*(u-16.64)/(88.03-16.64)-1
      settings: AttributesFormatString=%<Expr>
  Fcn5 : Fcn  Expr=2*(u-0)/(49-0)-1
      settings: AttributesFormatString=%<Expr>
  Fcn6 : Fcn  Expr=2*(u-40)/(46.18-0)-1
      settings: AttributesFormatString=%<Expr>
  Fcn7 : Fcn  Expr=2*(u-0.803)/(1.013-0.803)-1
      settings: AttributesFormatString=%<Expr>
  Mx1 : Mux  Inputs=5
  deg->SI : Gain  Gain=pi/180
  rad->deg : Gain
  Phi50 : Outport
  wires:
  deg->SI/1 -> Phi50/1
  Fcn5/1 -> Mx1/5
  DoE-Model PRESS 3.75/1 -> deg->SI/1
  Fcn7/1 -> Mx1/3
  0 ..1/1 -> Fcn7/1
  AFR/1 -> AFR->lambda/1
  AFR->lambda/1 -> 0 ..1/1  "VVTdeg"
  Fcn6/1 -> Mx1/4
  Fcn4/1 -> Mx1/2
  Fcn1/1 -> Mx1/1
  0 ..50/1 -> Fcn6/1
  SA/1 -> 0 .. 50/1
  0 .. 50/1 -> Fcn5/1
  Mx1/1 -> DoE-Model PRESS 3.75/1
  VVT/1 -> rad->deg/1
  KL/1 -> ->%/1
  N/1 -> 600 .. 6000/1
  ->%/1 -> 10 .. 100/1
  10 .. 100/1 -> Fcn4/1  "KL"
  600 .. 6000/1 -> Fcn1/1  "N"
  rad->deg/1 -> 0 ..50/1  "VVTdeg"

== system benchmark_model/ENGINE/engine_s/cylinders/cyl4/cyl/frame/Init_cyl_gas/capture_cyl_state/burnt_compsition/Subsystem ==
  af : Inport
  burnt : Inport  Port=2
  unburnt : Inport  Port=3
  C1 : Constant  Value=6
  C2 : Constant  Value=22
  Logical Operator : Logic  AllPortsSameDT=off  OutDataTypeStr=boolean
  Relational Operator : RelationalOperator  OutDataTypeStr=boolean  RndMeth=Nearest
  Relational Operator1 : RelationalOperator  Operator=<=  OutDataTypeStr=boolean  RndMeth=Nearest
  Switch : Switch  Threshold=0.5
  Out1 : Outport
  wires:
  unburnt/1 -> Switch/3
  Switch/1 -> Out1/1
  burnt/1 -> Switch/1
  af/1 -> Relational Operator/1, Relational Operator1/1
  C1/1 -> Relational Operator/2
  C2/1 -> Relational Operator1/2
  Relational Operator1/1 -> Logical Operator/2
  Relational Operator/1 -> Logical Operator/1
  Logical Operator/1 -> Switch/2

== system benchmark_model/ENGINE/engine_s/cylinders/cyl4/cyl/frame/ratio_burnt1/murnt_ratio/Phi050 DoE model/Subsystem ==
  note: SAmin changed from 0 to -15deg, PS1303131400
      |
      | N=((2*N-6599)./(5401));
      | KL=((2*KL-104.17)./(71.89));
      | LA=((2*LA-1.801)./(0.235));
      | VVT=((2*VVT-46.18)./(46.18));
      | SP=((2*SA-49)./(49));
      | EG=C02/interp(AL,CO2,14.5);
      | phi50-spark=exp(3.6636+0.16333.*N-0.2286.*KL+0.067945.*LA+0.058803.*VVT-0.1392.*SP+0.30732.*SP.^2-0.3238.*N.*SP);
  N : Inport
  KL : Inport  Port=2
  SA : Inport  Port=3
  VVT : Inport  Port=4
  AFR : Inport  Port=5
  ->% : Gain  Gain=100
  0 .. 50 : Saturate  UpperLimit=50  LowerLimit=-15  ZeroCross=off
      settings: AttributesFormatString=%<LowerLimit> .. %<UpperLimit>
  0 ..1 : Saturate  UpperLimit=1.013*0+2.0  LowerLimit=.803  ZeroCross=off
      settings: AttributesFormatString=%<LowerLimit> .. %<UpperLimit>
  0 ..50 : Saturate  UpperLimit=50  LowerLimit=0  ZeroCross=off
      settings: AttributesFormatString=%<LowerLimit> .. %<UpperLimit>
  10 .. 100 : Saturate  UpperLimit=88.03  LowerLimit=16.64  ZeroCross=off
      settings: AttributesFormatString=%<LowerLimit> .. %<UpperLimit>
  600 .. 6000 : Saturate  UpperLimit=6000  LowerLimit=599  ZeroCross=off
      settings: AttributesFormatString=%<LowerLimit> .. %<UpperLimit>
  AFR->lambda : Gain  Gain=1/14.5
  DoE-Model PRESS 3.75 : Fcn  Expr=exp(3.6636+0.16333*u(1)-0.2286*u(2)+0.067945*u(3)+0.058803*u(4)-0.1392*u(5)+0.30732*u(5)^2-0.3238*u(1)*u(5))
  Fcn1 : Fcn  Expr=2*(u-599)/(6000-599)-1
      settings: AttributesFormatString=%<Expr>
  Fcn4 : Fcn  Expr=2*(u-16.64)/(88.03-16.64)-1
      settings: AttributesFormatString=%<Expr>
  Fcn5 : Fcn  Expr=2*(u-0)/(49-0)-1
      settings: AttributesFormatString=%<Expr>
  Fcn6 : Fcn  Expr=2*(u-40)/(46.18-0)-1
      settings: AttributesFormatString=%<Expr>
  Fcn7 : Fcn  Expr=2*(u-0.803)/(1.013-0.803)-1
      settings: AttributesFormatString=%<Expr>
  Mx1 : Mux  Inputs=5
  deg->SI : Gain  Gain=pi/180
  rad->deg : Gain
  Phi50 : Outport
  wires:
  rad->deg/1 -> 0 ..50/1  "VVTdeg"
  600 .. 6000/1 -> Fcn1/1  "N"
  10 .. 100/1 -> Fcn4/1  "KL"
  ->%/1 -> 10 .. 100/1
  N/1 -> 600 .. 6000/1
  KL/1 -> ->%/1
  VVT/1 -> rad->deg/1
  Mx1/1 -> DoE-Model PRESS 3.75/1
  0 .. 50/1 -> Fcn5/1
  SA/1 -> 0 .. 50/1
  0 ..50/1 -> Fcn6/1
  Fcn1/1 -> Mx1/1
  Fcn4/1 -> Mx1/2
  Fcn6/1 -> Mx1/4
  AFR->lambda/1 -> 0 ..1/1  "VVTdeg"
  AFR/1 -> AFR->lambda/1
  0 ..1/1 -> Fcn7/1
  Fcn7/1 -> Mx1/3
  DoE-Model PRESS 3.75/1 -> deg->SI/1
  Fcn5/1 -> Mx1/5
  deg->SI/1 -> Phi50/1

== matlab function benchmark_model/ENGINE/engine_s/cylinders/cyl3/cyl/Energy_Int/dvol/func_d_cylvol(u,SPEC)/Embedded MATLAB Function1 ==
  settings: fimath=|
      | fimath(...
      | 'RoundMode', 'floor',...
      | 'OverflowMode', 'wrap',...
      | 'ProductMode', 'KeepLSB', 'ProductWordLength', 32,...
      | 'SumMode', 'KeepLSB', 'SumWordLength', 32,...
      | 'CastBeforeSum', false)
  data: u input; y output; SPEC input size=19
function y = func_d_cylvol(u,SPEC)
%SPEC=[ 1:NCYL;  2:BORE;  3:STROKE;  4:RCRK;  5:CNTL;
%       6:COMP;  7:mc;    8:Jc;      9:cc;   10:mr;
%      11:Jr;   12:cr;   13:mp;     14:cp;   15:a;
%      16:b;    17:y_bdc;18:y_tdc;  19:Jfw;];

BORE   = SPEC(2);
STROKE = SPEC(3);
r      = SPEC(4);
l      = SPEC(5);
COMP   = SPEC(6);

AREA = 0.25*pi*BORE^2;
VH = AREA*STROKE;
VT = VH/(COMP-1);

LL = l^2-(r*sin(u))^2;
y = AREA*r*sin(u)*(1.0+r*cos(u)/sqrt(LL));

== matlab function benchmark_model/ENGINE/engine_s/cylinders/cyl3/cyl/cal_cyl_state/cyl_vol ==
  settings: fimath=|
      | fimath(...
      | 'RoundMode', 'floor',...
      | 'OverflowMode', 'wrap',...
      | 'ProductMode', 'KeepLSB', 'ProductWordLength', 32,...
      | 'SumMode', 'KeepLSB', 'SumWordLength', 32,...
      | 'CastBeforeSum', false)
  data: u input; vol output; SPEC input size=19
function vol=func_cylvol(u,SPEC)
%SPEC=[ 1:NCYL;  2:BORE;  3:STROKE;  4:RCRK;  5:CNTL;
%       6:COMP;  7:mc;    8:Jc;      9:cc;   10:mr;
%      11:Jr;   12:cr;   13:mp;     14:cp;   15:a;
%      16:b;    17:y_bdc;18:y_tdc;  19:Jfw;];

   r    = SPEC(4);
   l    = SPEC(5);
   
   AREA = 0.25*pi*SPEC(2)*SPEC(2);
   VH = AREA*SPEC(3);
   VT = VH/(SPEC(6)-1);
   LL = l^2-(r*sin(u))^2;
   vol = VT+AREA*((r+l)-(r*cos(u)+sqrt(LL)));

== matlab function benchmark_model/ENGINE/engine_s/cylinders/cyl3/cyl/frame/ratio_burnt1/murnt_ratio/Embedded MATLAB Function ==
  data: u input; q output; Web input; Q output
function [q,Q]  = func_webC_s(u,Web)
% made by Alex on January 28th, 2010
%   y: burnt ratio
%   u: crank angle that takes 0 at the compression TDC
% Web: parameters
%
WebA = Web(1);
WebM = Web(2);
WebT = Web(3);
WebS = Web(4);
WWebs = pi-WebS;

uu = mod(u,4*pi)-WWebs;
if (uu>0)   
    q = 1.0/WebT*(WebM+1.0)*WebA*(uu/WebT)^WebM*...
          exp(-WebA*(uu/WebT)^(WebM+1.0));
    Q = 1-exp(-WebA*(uu/WebT)^(WebM+1.0));
else
    q = 0;
    Q = 0;
end

== stateflow chart benchmark_model/ENGINE/engine_s/cylinders/cyl3/cyl/unburnt_gass/init&trig/qChart ==
  state A/
    exit:
    sl_out1=sl_in1;
    sl_out2=sl_in2;
    sl_out3=sl_in3;
    sl_out4=sl_in4;
    sl_out5=sl_in5;
    sl_out6=sl_in6;
    sl_out7=sl_in7;
  (default) -> A : {sl_out1=sl_in1;
      |  sl_out2=sl_in2;
      |  sl_out3=sl_in3;
      |  sl_out4=sl_in4;
      |  sl_out5=sl_in5;
      |  sl_out6=sl_in6;
      |  sl_out7=sl_in7;
      | }
  A -> A : event
  data: sl_in1 input; sl_out1 output double =NHC; sl_in2 input; sl_in3 input; sl_in4 input; sl_in5 input; sl_in6 input; sl_in7 input; sl_out2 output double =NCO2; sl_out3 output double =NCO; sl_out4 output double =NO2; sl_out5 output double =NH2; sl_out6 output double =NH2O; sl_out7 output double =NN2
  events: event input RISING_EDGE_EVENT

== matlab function benchmark_model/ENGINE/engine_s/cylinders/cyl3/ex_valve/cal_flow ==
  data: area input; fen output; inlet input; c_in input; outlet input; c_out input; fml output; WOM input
function [fen,fml] = func_nozzle(area,inlet,c_in,outlet,c_out,WOM) 
% made by Alex on February 3rd, 2010
% This program calculates the flow rate through the nozzle 
% under the assamption that the mass, the energy and the mometum
% are conserved between the inlet and the outlet flows.
%
% The inlet and the outlet are connected with the sign convention 
% of the calculated flow. The sign of the flow from th einlet and 
% the outlet is positive.
%
% inlet(1):pressure 
% inlet(2):density
% inlet(3):weight of molecule
% inlet(4):degree of freedom
% outlet(1):pressure 
% outlet(2):density
% outlet(3):weight of molecule
% outlet(4):degree of freedom

y = zeros(8,1); % modified 

du = inlet(1);
pu = inlet(2);
mu = inlet(3);
fu = inlet(4);
dd = outlet(1);
pd = outlet(2);
if dd<0
    dd=0;
end
md = outlet(3);
fd = outlet(4);
AR = area;

if (pu >= pd)
    rp = pd/pu;
    k = (fu + 2.0)/fu;
    crp = 1.0/(k + 1.0);
    A = AR*sqrt(abs((k + 1.0)/(2.0*k)*pu*du));
    B = sqrt((k/(k + 1.0))^2 - (0.99 - 1.0/(k + 1.0))^2);
    C = -(0.99 - 1.0/(k + 1.0))/B;
    a = (C*0.01 - B)/(2.0*0.01^3);
    c = C - 3.0*a*0.01^2;
    if (rp >= 0.99)
      fms = A*(a*(1.0 - rp)^3 + c*(1.0 - rp));
    else
      if (rp >= crp)
        R = (k/(k + 1.0))^2 - (rp - 1.0/(k + 1.0))^2;
        if (R < 0)
          R = 0;
        end
        fms = A*sqrt(R);
      else
        fms = A*k/(k + 1.0);
      end
    end
    fen = fms*(fu + 2.0)/2.0*pu/du;
    Ma = WOM'*c_in;
    fml = c_in*fms/Ma;
  else
    rp = pu/pd;
    k = (fd + 2.0)/fd;
    crp = 1.0/(k + 1.0);
    A = AR*sqrt((k + 1.0)/(2.0*k)*pd*dd);
    B = sqrt((k/(k + 1.0))^2 - (0.99 - 1.0/(k + 1.0))^2);
    C = (0.99 - 1.0/(k + 1.0))/B;
    a = (C*0.01 - B)/(2.0*0.01^3);
    c = C - 3.0*a*0.01^2;
    if (rp >= 0.99)
      fms = -A*(a*(1.0 - rp)^3 + c*(1.0 - rp));
    else
      if (rp >= crp)
        R = (k/(k + 1.0))^2 - (rp - 1.0/(k + 1.0))^2;
        if (R < 0)
          R = 0;
        end
        fms = -A*sqrt(R);
      else
        fms = -A*k/(k + 1.0);
      end
    end
    fen = fms*(fd + 2.0)/2.0*pd/dd;
    Ma = WOM'*c_out;
    fml = c_out*fms/Ma;
end
if isnan(fen)
       fen=0;
end

== matlab function benchmark_model/ENGINE/engine_s/cylinders/cyl3/in_valve/cal_flow ==
  data: area input; fen output; inlet input; c_in input; outlet input; c_out input; fml output; fms output; WOM input
function [fen,fml,fms] = func_nozzle(area,inlet,c_in,outlet,c_out,WOM) 
% made by Alex on February 3rd, 2010
% This program calculates the flow rate through the nozzle 
% under the assamption that the mass, the energy and the mometum
% are conserved between the inlet and the outlet flows.
%
% The inlet and the outlet are connected with the sign convention 
% of the calculated flow. The sign of the flow from th einlet and 
% the outlet is positive.
%
% inlet(1):pressure 
% inlet(2):density
% inlet(3):weight of molecule
% inlet(4):degree of freedom
% outlet(1):pressure 
% outlet(2):density
% outlet(3):weight of molecule
% outlet(4):degree of freedom

y = zeros(8,1); % modified 

du = inlet(1);
pu = inlet(2);
mu = inlet(3);
fu = inlet(4);
dd = outlet(1);
if dd<0
    dd=1e-9
end
pd = outlet(2);
md = outlet(3);
fd = outlet(4);
AR = area;

if (pu >= pd)
    rp = pd/pu;
    k = (fu + 2.0)/fu;
    crp = 1.0/(k + 1.0);
    A = AR*sqrt((k + 1.0)/(2.0*k)*pu*du);
    B = sqrt((k/(k + 1.0))^2 - (0.99 - 1.0/(k + 1.0))^2);
    C = -(0.99 - 1.0/(k + 1.0))/B;
    a = (C*0.01 - B)/(2.0*0.01^3);
    c = C - 3.0*a*0.01^2;
    if (rp >= 0.99)
      fms = A*(a*(1.0 - rp)^3 + c*(1.0 - rp));
    else
      if (rp >= crp)
        R = (k/(k + 1.0))^2 - (rp - 1.0/(k + 1.0))^2;
        if (R < 0)
          R = 0;
        end
        fms = A*sqrt(R);
      else
        fms = A*k/(k + 1.0);
      end
    end
    fen = fms*(fu + 2.0)/2.0*pu/du;
    Ma = WOM'*c_in;
    fml = c_in*fms/Ma;
  else
    rp = pu/pd;
    k = (fd + 2.0)/fd;
    crp = 1.0/(k + 1.0);
    A = AR*sqrt((k + 1.0)/(2.0*k)*pd*dd);
    B = sqrt((k/(k + 1.0))^2 - (0.99 - 1.0/(k + 1.0))^2);
    C = (0.99 - 1.0/(k + 1.0))/B;
    a = (C*0.01 - B)/(2.0*0.01^3);
    c = C - 3.0*a*0.01^2;
    if (rp >= 0.99)
      fms = -A*(a*(1.0 - rp)^3 + c*(1.0 - rp));
    else
      if (rp >= crp)
        R = (k/(k + 1.0))^2 - (rp - 1.0/(k + 1.0))^2;
        if (R < 0)
          R = 0;
        end
        fms = -A*sqrt(R);
      else
        fms = -A*k/(k + 1.0);
      end
    end
    fen = fms*(fd + 2.0)/2.0*pd/dd;
    Ma = WOM'*c_out;
    fml = c_out*fms/Ma;
end
if isnan(fen)
    fen=0;
end

== matlab function benchmark_model/ENGINE/engine_s/cylinders/cyl4/cyl/Energy_Int/dvol/func_d_cylvol(u,SPEC)/Embedded MATLAB Function1 ==
  settings: fimath=|
      | fimath(...
      | 'RoundMode', 'floor',...
      | 'OverflowMode', 'wrap',...
      | 'ProductMode', 'KeepLSB', 'ProductWordLength', 32,...
      | 'SumMode', 'KeepLSB', 'SumWordLength', 32,...
      | 'CastBeforeSum', false)
  data: u input; y output; SPEC input size=19
function y = func_d_cylvol(u,SPEC)
%SPEC=[ 1:NCYL;  2:BORE;  3:STROKE;  4:RCRK;  5:CNTL;
%       6:COMP;  7:mc;    8:Jc;      9:cc;   10:mr;
%      11:Jr;   12:cr;   13:mp;     14:cp;   15:a;
%      16:b;    17:y_bdc;18:y_tdc;  19:Jfw;];

BORE   = SPEC(2);
STROKE = SPEC(3);
r      = SPEC(4);
l      = SPEC(5);
COMP   = SPEC(6);

AREA = 0.25*pi*BORE^2;
VH = AREA*STROKE;
VT = VH/(COMP-1);

LL = l^2-(r*sin(u))^2;
y = AREA*r*sin(u)*(1.0+r*cos(u)/sqrt(LL));

== matlab function benchmark_model/ENGINE/engine_s/cylinders/cyl4/cyl/cal_cyl_state/cyl_vol ==
  settings: fimath=|
      | fimath(...
      | 'RoundMode', 'floor',...
      | 'OverflowMode', 'wrap',...
      | 'ProductMode', 'KeepLSB', 'ProductWordLength', 32,...
      | 'SumMode', 'KeepLSB', 'SumWordLength', 32,...
      | 'CastBeforeSum', false)
  data: u input; vol output; SPEC input size=19
function vol=func_cylvol(u,SPEC)
%SPEC=[ 1:NCYL;  2:BORE;  3:STROKE;  4:RCRK;  5:CNTL;
%       6:COMP;  7:mc;    8:Jc;      9:cc;   10:mr;
%      11:Jr;   12:cr;   13:mp;     14:cp;   15:a;
%      16:b;    17:y_bdc;18:y_tdc;  19:Jfw;];

   r    = SPEC(4);
   l    = SPEC(5);
   
   AREA = 0.25*pi*SPEC(2)*SPEC(2);
   VH = AREA*SPEC(3);
   VT = VH/(SPEC(6)-1);
   LL = l^2-(r*sin(u))^2;
   vol = VT+AREA*((r+l)-(r*cos(u)+sqrt(LL)));

== matlab function benchmark_model/ENGINE/engine_s/cylinders/cyl4/cyl/frame/ratio_burnt1/murnt_ratio/Embedded MATLAB Function ==
  data: u input; q output; Web input; Q output
function [q,Q]  = func_webC_s(u,Web)
% made by Alex on January 28th, 2010
%   y: burnt ratio
%   u: crank angle that takes 0 at the compression TDC
% Web: parameters
%
WebA = Web(1);
WebM = Web(2);
WebT = Web(3);
WebS = Web(4);
WWebs = pi-WebS;

uu = mod(u,4*pi)-WWebs;
if (uu>0)   
    q = 1.0/WebT*(WebM+1.0)*WebA*(uu/WebT)^WebM*...
          exp(-WebA*(uu/WebT)^(WebM+1.0));
    Q = 1-exp(-WebA*(uu/WebT)^(WebM+1.0));
else
    q = 0;
    Q = 0;
end

== matlab function benchmark_model/ENGINE/engine_s/cylinders/cyl1/cyl/Energy_Int/dvol/func_d_cylvol(u,SPEC)/Embedded MATLAB Function1 ==
  settings: fimath=|
      | fimath(...
      | 'RoundMode', 'floor',...
      | 'OverflowMode', 'wrap',...
      | 'ProductMode', 'KeepLSB', 'ProductWordLength', 32,...
      | 'SumMode', 'KeepLSB', 'SumWordLength', 32,...
      | 'CastBeforeSum', false)
  data: u input; y output; SPEC input size=19
function y = func_d_cylvol(u,SPEC)
%SPEC=[ 1:NCYL;  2:BORE;  3:STROKE;  4:RCRK;  5:CNTL;
%       6:COMP;  7:mc;    8:Jc;      9:cc;   10:mr;
%      11:Jr;   12:cr;   13:mp;     14:cp;   15:a;
%      16:b;    17:y_bdc;18:y_tdc;  19:Jfw;];

BORE   = SPEC(2);
STROKE = SPEC(3);
r      = SPEC(4);
l      = SPEC(5);
COMP   = SPEC(6);

AREA = 0.25*pi*BORE^2;
VH = AREA*STROKE;
VT = VH/(COMP-1);

LL = l^2-(r*sin(u))^2;
y = AREA*r*sin(u)*(1.0+r*cos(u)/sqrt(LL));

== matlab function benchmark_model/ENGINE/engine_s/cylinders/cyl1/cyl/cal_cyl_state/cyl_vol ==
  settings: fimath=|
      | fimath(...
      | 'RoundMode', 'floor',...
      | 'OverflowMode', 'wrap',...
      | 'ProductMode', 'KeepLSB', 'ProductWordLength', 32,...
      | 'SumMode', 'KeepLSB', 'SumWordLength', 32,...
      | 'CastBeforeSum', false)
  data: u input; vol output; SPEC input size=19
function vol=func_cylvol(u,SPEC)
%SPEC=[ 1:NCYL;  2:BORE;  3:STROKE;  4:RCRK;  5:CNTL;
%       6:COMP;  7:mc;    8:Jc;      9:cc;   10:mr;
%      11:Jr;   12:cr;   13:mp;     14:cp;   15:a;
%      16:b;    17:y_bdc;18:y_tdc;  19:Jfw;];

   r    = SPEC(4);
   l    = SPEC(5);
   
   AREA = 0.25*pi*SPEC(2)*SPEC(2);
   VH = AREA*SPEC(3);
   VT = VH/(SPEC(6)-1);
   LL = l^2-(r*sin(u))^2;
   vol = VT+AREA*((r+l)-(r*cos(u)+sqrt(LL)));

== stateflow chart benchmark_model/ENGINE/engine_s/cylinders/cyl4/cyl/unburnt_gass/init&trig/qChart ==
  state A/
    exit:
    sl_out1=sl_in1;
    sl_out2=sl_in2;
    sl_out3=sl_in3;
    sl_out4=sl_in4;
    sl_out5=sl_in5;
    sl_out6=sl_in6;
    sl_out7=sl_in7;
  (default) -> A : {sl_out1=sl_in1;
      |  sl_out2=sl_in2;
      |  sl_out3=sl_in3;
      |  sl_out4=sl_in4;
      |  sl_out5=sl_in5;
      |  sl_out6=sl_in6;
      |  sl_out7=sl_in7;
      | }
  A -> A : event
  data: sl_in1 input; sl_out1 output double =NHC; sl_in2 input; sl_in3 input; sl_in4 input; sl_in5 input; sl_in6 input; sl_in7 input; sl_out2 output double =NCO2; sl_out3 output double =NCO; sl_out4 output double =NO2; sl_out5 output double =NH2; sl_out6 output double =NH2O; sl_out7 output double =NN2
  events: event input RISING_EDGE_EVENT

== matlab function benchmark_model/ENGINE/engine_s/cylinders/cyl1/cyl/frame/ratio_burnt1/murnt_ratio/Embedded MATLAB Function ==
  data: u input; q output; Web input; Q output
function [q,Q]  = func_webC_s(u,Web)
% made by Alex on January 28th, 2010
%   y: burnt ratio
%   u: crank angle that takes 0 at the compression TDC
% Web: parameters
%
WebA = Web(1);
WebM = Web(2);
WebT = Web(3);
WebS = Web(4);
WWebs = pi-WebS;

uu = mod(u,4*pi)-WWebs;
if (uu>0)   
    q = 1.0/WebT*(WebM+1.0)*WebA*(uu/WebT)^WebM*...
          exp(-WebA*(uu/WebT)^(WebM+1.0));
    Q = 1-exp(-WebA*(uu/WebT)^(WebM+1.0));
else
    q = 0;
    Q = 0;
end

== stateflow chart benchmark_model/ENGINE/engine_s/cylinders/cyl1/cyl/unburnt_gass/init&trig/qChart ==
  state A/
    exit:
    sl_out1=sl_in1;
    sl_out2=sl_in2;
    sl_out3=sl_in3;
    sl_out4=sl_in4;
    sl_out5=sl_in5;
    sl_out6=sl_in6;
    sl_out7=sl_in7;
  (default) -> A : {sl_out1=sl_in1;
      |  sl_out2=sl_in2;
      |  sl_out3=sl_in3;
      |  sl_out4=sl_in4;
      |  sl_out5=sl_in5;
      |  sl_out6=sl_in6;
      |  sl_out7=sl_in7;
      | }
  A -> A : event
  data: sl_in1 input; sl_out1 output double =NHC; sl_in2 input; sl_in3 input; sl_in4 input; sl_in5 input; sl_in6 input; sl_in7 input; sl_out2 output double =NCO2; sl_out3 output double =NCO; sl_out4 output double =NO2; sl_out5 output double =NH2; sl_out6 output double =NH2O; sl_out7 output double =NN2
  events: event input RISING_EDGE_EVENT
